simulink model "Project_2_Kinematic_Model"  (R2025a)
settings: Solver=VariableStepAuto  StartTime=0.0  StopTime=10.0  RelTol=1e-3
settings Model: Creator=jr843  LastModifiedBy=jr843

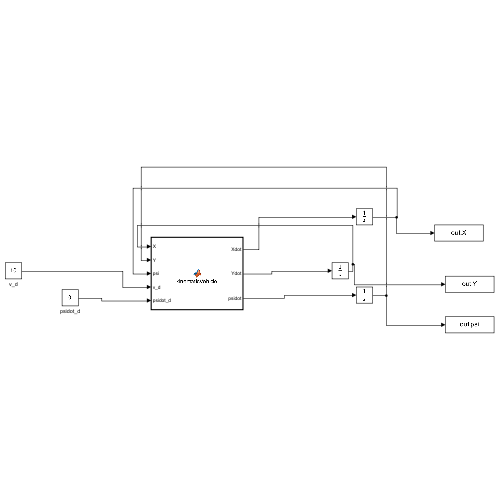
[thumbnail: Simulink's stored preview of the top-level diagram]
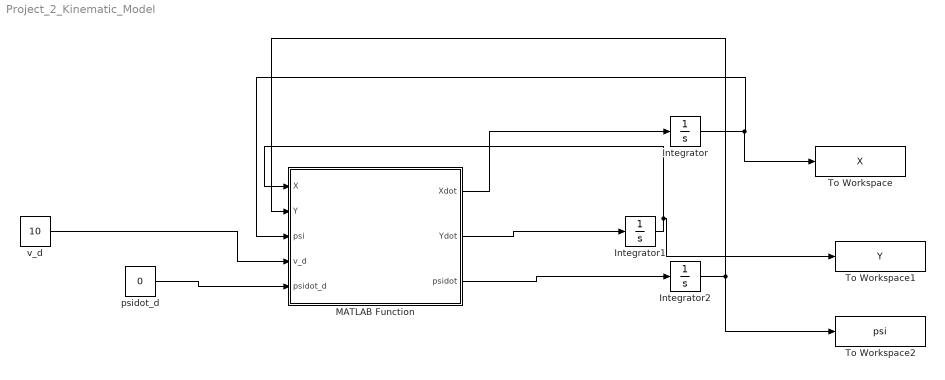
== system Project_2_Kinematic_Model ==
  Integrator : Integrator
  Integrator1 : Integrator
  Integrator2 : Integrator
  MATLAB Function : MATLAB Function  TreatAsAtomicUnit=on
  To Workspace : ToWorkspace  VariableName=X  SaveFormat=Timeseries  SampleTime=-1
  To Workspace1 : ToWorkspace  VariableName=Y  SaveFormat=Timeseries  SampleTime=-1
  To Workspace2 : ToWorkspace  VariableName=psi  SaveFormat=Timeseries  SampleTime=-1
  psidot_d : Constant  Value=0
  v_d : Constant  Value=10
  wires:
  v_d/1 -> MATLAB Function/4(v_d)
  psidot_d/1 -> MATLAB Function/5(psidot_d)
  MATLAB Function/2(Ydot) -> Integrator1/1
  MATLAB Function/1(Xdot) -> Integrator/1
  MATLAB Function/3(psidot) -> Integrator2/1
  Integrator/1 -> To Workspace/1, MATLAB Function/3(psi)
  Integrator2/1 -> To Workspace2/1, MATLAB Function/2(Y)
  Integrator1/1 -> To Workspace1/1, MATLAB Function/1(X)

== matlab function Project_2_Kinematic_Model/MATLAB Function ==
  data: X input; Y input; psi input; Xdot output; v_d input; Ydot output; psidot_d input; psidot output
function [Xdot, Ydot, psidot] = kinematicVehicle(X, Y, psi, v_d, psidot_d)
    Xdot = v_d * cos(psi);
    Ydot = v_d * sin(psi);
    psidot = psidot_d;
end
